simulink model "untitled"  (R2022b)
settings: Solver=FixedStepDiscrete  StartTime=0.0  StopTime=10.0  RelTol=1e-3
settings Model: DataDictionary=test.sldd  Creator=15801  LastModifiedBy=15801
settings OptimizationCC: DefaultParameterBehavior=Inlined  EnhancedBackFolding=on  PassReuseOutputArgsAs=Individual arguments  ZeroExternalMemoryAtStartup=off  ZeroInternalMemoryAtStartup=off  OptimizeBlockOrder=speed  DifferentSizesBufferReuse=on  OptimizationCustomize=off  EfficientTunableParamExpr=on
settings DebuggingCC: ParameterTunabilityLossMsg=error
settings SFSimCC: MATLABDynamicMemAlloc=off
settings RTWCC: Description=Embedded Coder  SystemTargetFile=ert.tlc  TemplateMakefile=ert_default_tmf
settings CodeAppCC: ForceParamTrailComments=on  IgnoreCustomStorageClasses=off  OperatorAnnotations=on  SimulinkDataObjDesc=on  SFDataObjDesc=on  InsertBlockDesc=on
settings ERTTargetCC: TargetLangStandard=C99 (ISO)  GenerateSampleERTMain=on  InlinedParameterPlacement=NonHierarchical  ERTCustomFileTemplate=example_file_process.tlc

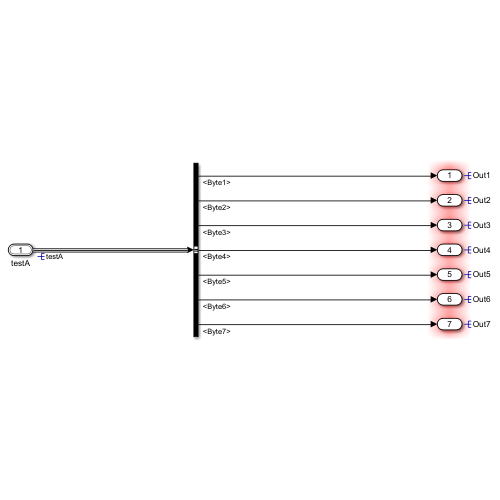
[thumbnail: Simulink's stored preview of the top-level diagram]
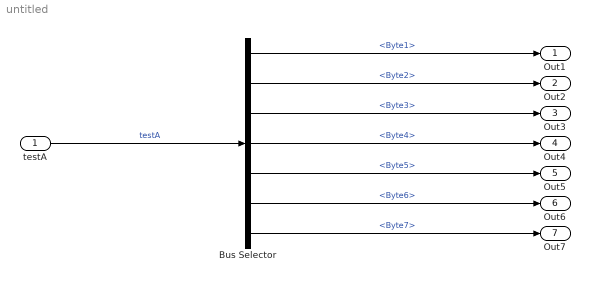
== system untitled ==
  testA : Inport  OutDataTypeStr=Bus: test
  Bus Selector : BusSelector  OutputSignals=Byte1,Byte2,Byte3,Byte4,Byte5,Byte6,Byte7
  Out1 : Outport  SignalName=Out1
      settings: MustResolveToSignalObject=on
  Out2 : Outport  Port=2  SignalName=Out2
      settings: MustResolveToSignalObject=on
  Out3 : Outport  Port=3  SignalName=Out3
      settings: MustResolveToSignalObject=on
  Out4 : Outport  Port=4  SignalName=Out4
      settings: MustResolveToSignalObject=on
  Out5 : Outport  Port=5  SignalName=Out5
      settings: MustResolveToSignalObject=on
  Out6 : Outport  Port=6  SignalName=Out6
      settings: MustResolveToSignalObject=on
  Out7 : Outport  Port=7  SignalName=Out7
      settings: MustResolveToSignalObject=on
  wires:
  testA/1 -> Bus Selector/1  "testA"
  Bus Selector/1 -> Out1/1  "<Byte1>"
  Bus Selector/2 -> Out2/1  "<Byte2>"
  Bus Selector/3 -> Out3/1  "<Byte3>"
  Bus Selector/4 -> Out4/1  "<Byte4>"
  Bus Selector/5 -> Out5/1  "<Byte5>"
  Bus Selector/6 -> Out6/1  "<Byte6>"
  Bus Selector/7 -> Out7/1  "<Byte7>"
